simulink model "PRIMER3"  (R2018a)
settings: Solver=VariableStepAuto  StartTime=0.0  StopTime=100  RelTol=1e-3
values from neighbouring files (symbols this model uses):
  q0 = -1.1901    [AV10_ZADACHA1.m]    (also in AV9_PRIMER2_VREDNOSTI.m = -62.3782; AV9_PRIMER4.m = 1.9573; AV9_PRIMER5.m = 1.8649; AV_10_PRIMER1.m = 1.512)
  q1 = 0.8945    [AV10_ZADACHA1.m]    (also in AV9_PRIMER2_VREDNOSTI.m = 122.0694; AV9_PRIMER4.m = -1.6594; AV9_PRIMER5.m = -1.8649; AV_10_PRIMER1.m = -1.423)
  q2 = -0.2805    [AV10_ZADACHA1.m]    (also in AV9_PRIMER2_VREDNOSTI.m = -59.9743; AV9_PRIMER4.m = 0.6675; AV9_PRIMER5.m = 0.2403; AV_10_PRIMER1.m = 0.44)
  T0 = 16    [A12-2 Pol nula ponistuvacki upravuvac primeri 1 i 2.m]    (also in AV9_PRIMER2_VREDNOSTI.m = 160; AV_8_PRIMER3.m = 1)
settings Model: Creator=DD  LastModifiedBy=DD

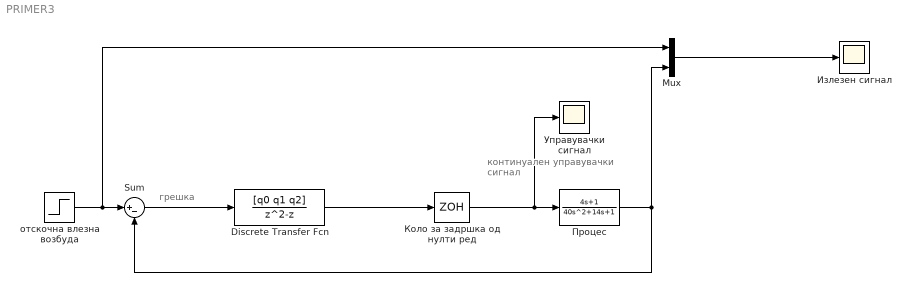
== system PRIMER3 ==
  note: континуален управувачки сигнал
  note: грешка
  " Процес " : TransferFcn  Numerator=[4 1]  Denominator=[40 14 1]
  Discrete Transfer Fcn : DiscreteTransferFcn  Numerator=[q0 q1 q2]  Denominator=[1 -1 0]  SampleTime=T0
  Mux : Mux  Inputs=2
  Sum : Sum  Inputs=|+-
  Излезен сигнал : Scope
  "Коло за задршка од нулти ред " : ZeroOrderHold  SampleTime=-1
  "Управувачки сигнал " : Scope
  отскочна влезна возбуда : Step  SampleTime=0
  wires:
  Discrete Transfer Fcn/1 -> "Коло за задршка од нулти ред "/1
  "Коло за задршка од нулти ред "/1 -> "Управувачки сигнал "/1, " Процес "/1
  Sum/1 -> Discrete Transfer Fcn/1
  " Процес "/1 -> Mux/2, Sum/2
  Mux/1 -> Излезен сигнал/1
  отскочна влезна возбуда/1 -> Mux/1, Sum/1
